simulink model "model3"  (R2022a)
settings: Solver=FixedStepAuto  StartTime=0.0  StopTime=5  FixedStep=1e-5  RelTol=1e-3
PreLoadFcn:
  | m = 3.600;     % kg
  | k = 400;    % N/m
  | b = 10;      % Ns/m
  | x0=1; %m
settings Model: Creator=whatastarrynight  LastModifiedBy=whatastarrynight

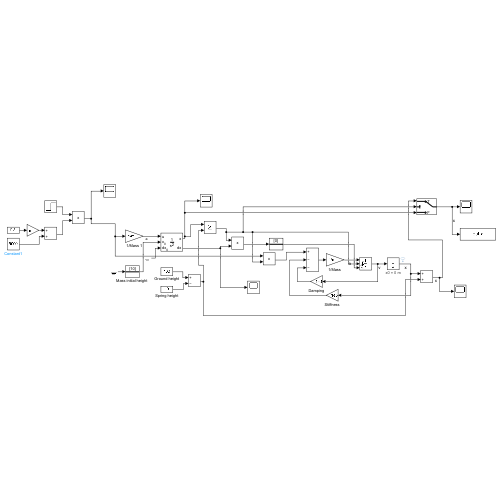
[thumbnail: Simulink's stored preview of the top-level diagram]
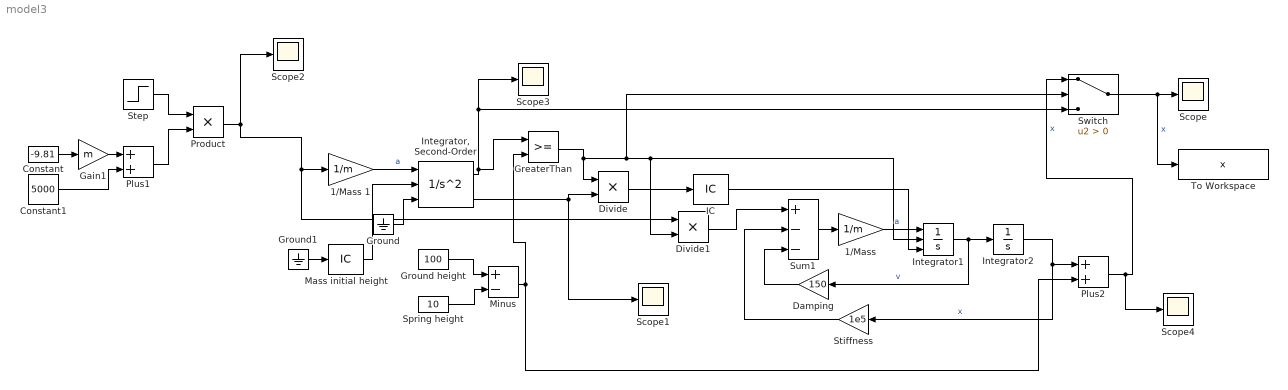
== system model3 ==
  "1/Mass " : Gain  Gain=1/m  SaturateOnIntegerOverflow=on  OutDataTypeStr=Inherit: Same as input  ParamDataTypeStr=Inherit: Same as input
  1/Mass 1 : Gain  Gain=1/m  SaturateOnIntegerOverflow=on  OutDataTypeStr=Inherit: Same as input  ParamDataTypeStr=Inherit: Same as input
  Constant : Constant  Value=-9.81
  Constant1 : Constant  Value=5000
  Damping : Gain  Gain=150  SaturateOnIntegerOverflow=on  OutDataTypeStr=Inherit: Same as input  ParamDataTypeStr=Inherit: Same as input
  Divide : Product  Inputs=**
  Divide1 : Product  Inputs=**
  Gain1 : Gain  Gain=m
  GreaterThan : RelationalOperator  OutDataTypeStr=boolean  RndMeth=Simplest  InputSameDT=off
  Ground : Ground
  Ground height : Constant  Value=100
  Ground1 : Ground
  IC : InitialCondition  Value=0
  "Integrator, Second-Order" : SecondOrderIntegrator  ICSourceX=external  ICX=5.  ICSourceDXDT=external
  Integrator1 : Integrator  ExternalReset=rising  InitialConditionSource=external
  Integrator2 : Integrator
      settings: AttributesFormatString=x0 = %<InitialCondition> m
  "Mass initial height " : InitialCondition  Value=10
  Minus : Sum  Inputs=+-
  Plus1 : Sum
  Plus2 : Sum
  Product : Product
  Scope{,1..4} (5 alike) : Scope
  Spring height : Constant  Value=10
  Step : Step  Time=2  SampleTime=0
  Stiffness : Gain  Gain=1e5  SaturateOnIntegerOverflow=on  OutDataTypeStr=Inherit: Same as input  ParamDataTypeStr=Inherit: Same as input
  Sum1 : Sum  Inputs=+--  InputSameDT=on  SaturateOnIntegerOverflow=on  OutDataTypeStr=Inherit: Same as first input
  Switch : Switch  Criteria=u2 > Threshold  SaturateOnIntegerOverflow=off  InputSameDT=off
  To Workspace : ToWorkspace  VariableName=x  SaveFormat=Timeseries  SampleTime=-1
  wires:
  Stiffness/1 -> Sum1/2
  Sum1/1 -> "1/Mass "/1
  Integrator2/1 -> Plus2/1, Stiffness/1  "x"
  "1/Mass "/1 -> Integrator1/1  "a"
  Damping/1 -> Sum1/3
  Integrator1/1 -> Integrator2/1, Damping/1  "v"
  Constant/1 -> Gain1/1
  "Integrator, Second-Order"/1 -> GreaterThan/1, Scope3/1, Switch/3
  "Integrator, Second-Order"/2 -> Divide/2, Scope1/1
  Divide/1 -> IC/1
  IC/1 -> Integrator1/3
  Divide1/1 -> Sum1/1
  Product/1 -> Divide1/1, 1/Mass 1/1, Scope2/1
  Gain1/1 -> Plus1/1
  Constant1/1 -> Plus1/2
  1/Mass 1/1 -> "Integrator, Second-Order"/1  "a"
  Ground height/1 -> Minus/1
  Spring height/1 -> Minus/2
  Ground1/1 -> "Mass initial height "/1
  Minus/1 -> GreaterThan/2, Plus2/2
  Plus2/1 -> Scope4/1, Switch/1  "x"
  Switch/1 -> To Workspace/1, Scope/1  "x"
  Step/1 -> Product/1
  Plus1/1 -> Product/2
  Ground/1 -> "Integrator, Second-Order"/3
  "Mass initial height "/1 -> "Integrator, Second-Order"/2
  GreaterThan/1 -> Divide/1, Switch/2, Divide1/2, Integrator1/2
